simulink model "MPPT_Fuzzy"  (R2021b)
settings: Solver=ode45  StartTime=0.0  StopTime=1  FixedStep=1e-5  MaxStep=1e-4  RelTol=10e-4  EnableMultiTasking=on
libraries: spsSeriesRLCBranchLib x6, spsStairGeneratorLib x4, spsIdealSwitchLib x3, spsDiodeLib x1, fuzblock x1, powerlib_extras x1, spsGroundLib x1, spsIGBTDiodeLib x1, spsCurrentMeasurementLib x1, spsVoltageMeasurementLib x1, spsPVArrayLib x1, spsPWMGeneratorDCDCLib x1
settings Model: Creator=Administrator  LastModifiedBy=Madesh
settings SolverCC: AlgebraicLoopSolver=TrustRegion
settings DataIOCC: LimitDataPoints=on  SaveFormat=Array  SignalLoggingSaveFormat=ModelDataLogs  ReturnWorkspaceOutputs=off
settings OptimizationCC: ExpressionDepthLimit=2147483647  LifeSpan=inf
settings DebuggingCC: UnderspecifiedInitializationDetection=Classic  MergeDetectMultiDrivingBlocksExec=none  SolverPrmCheckMsg=warning  FcnCallInpInsideContextMsg=warning  StateNameClashWarn=warning  SFUnexpectedBacktrackingDiag=warning  SFNoUnconditionalDefaultTransitionDiag=warning  SFExecutionAtInitializationDiag=none  SFMachineParentedDataDiag=warning  ArithmeticOperatorsInVariantConditions=warning
settings HardwareCC: ProdBitPerPointer=32  ProdBitPerSizeT=32  ProdBitPerPtrDiffT=32  ProdLargestAtomicFloat=None  ProdIntDivRoundTo=Undefined  ProdEndianess=Unspecified  ProdWordSize=32  ProdHWDeviceType=32-bit Generic
settings ModelReferenceCC: PropagateSignalLabelsOutOfModel=off
settings SFSimCC: SimUseLocalCustomCode=off  CustomCodeUndefinedFunction=UseInterfaceOnly
settings RTWCC: RTWUseLocalCustomCode=off
settings CodeAppCC: StateflowObjectComments=on
settings GRTTargetCC: TargetLangStandard=C89/C90 (ANSI)  CombineOutputUpdateFcns=off  GRTInterface=on
settings ConfigComp: CovMetricSettings=dw  CovSaveCumulativeToWorkspaceVar=on  CovSaveSingleToWorkspaceVar=on  CovExternalEMLEnable=off
settings SimscapeCC: SimscapeNormalizeSystem=off

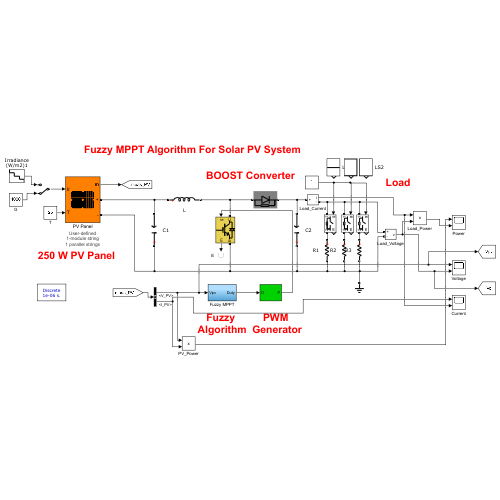
[thumbnail: Simulink's stored preview of the top-level diagram]
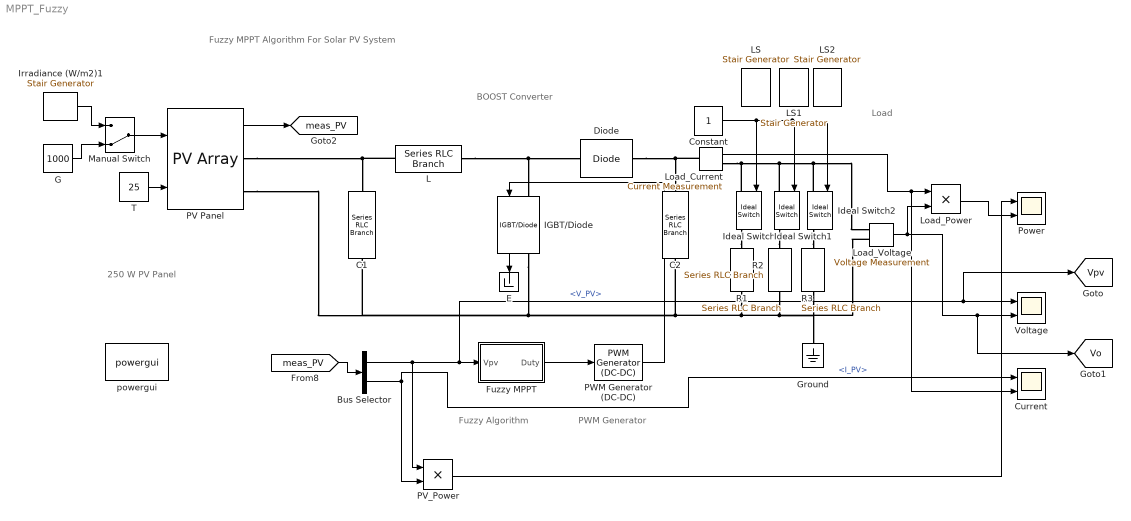
== system MPPT_Fuzzy ==
  note: Load
  note: Fuzzy MPPT Algorithm For Solar PV System
  note: BOOST Converter
  note: 250 W PV Panel
  note: Fuzzy
      | Algorithm
  note: PWM
      | Generator
  Bus Selector : BusSelector  OutputSignals=V_PV,I_PV
  C1 : spsSeriesRLCBranchLib/Series RLC Branch  LConnTagsString=__new0  RConnTagsString=__new0  BranchType=C  Resistance=1  Inductance=1e-3  SetiL0=off  InitialCurrent=0  Capacitance=100e-6  Setx0=off  InitialVoltage=0  Measurements=None
  C2 : spsSeriesRLCBranchLib/Series RLC Branch  LConnTagsString=__new0  RConnTagsString=__new0  BranchType=C  Resistance=1  Inductance=1e-3  SetiL0=off  InitialCurrent=0  Capacitance=100e-6  Setx0=off  InitialVoltage=0  Measurements=None
  Constant : Constant
  Current : Scope  NumInputPorts=2
  Diode : spsDiodeLib/Diode  Ron=0.001  Lon=0  Vf=0.8  IC=0  UseSnubber=off  Rs=500  Cs=250e-9  Measurements=off
  E : Terminator
  Fuzzy MPPT : Subsystem
  G : Constant  Value=1000
  Ground : spsGroundLib/Ground  LConnTagsString=a
  IGBT/Diode : spsIGBTDiodeLib/IGBT//Diode  Ron=1e-3  Rs=1e5  Cs=inf  Measurements=on
  Ideal Switch : spsIdealSwitchLib/Ideal Switch  Ron=0.001  Lon=0  IC=0  Rs=1e5  Cs=inf  Measurements=on
  Ideal Switch1 : spsIdealSwitchLib/Ideal Switch  Ron=0.001  Lon=0  IC=0  Rs=1e5  Cs=inf  Measurements=on
  Ideal Switch2 : spsIdealSwitchLib/Ideal Switch  Ron=0.001  Lon=0  IC=0  Rs=1e5  Cs=inf  Measurements=on
  Irradiance (W/m2)1 : spsStairGeneratorLib/Stair Generator  t=[0, 0.2 , 0.4 , 0.6, 0.8]  e=[1,0.8,0.6,0.4, 0.2]*1000  Ts=0.0001
  L : spsSeriesRLCBranchLib/Series RLC Branch  LConnTagsString=__new0  RConnTagsString=__new0  BranchType=L  Resistance=1  Inductance=3e-3  SetiL0=off  InitialCurrent=0  Capacitance=1e-6  Setx0=off  InitialVoltage=0  Measurements=None
  LS : spsStairGeneratorLib/Stair Generator  t=[0, 0.3]  e=[1, 0]  Ts=0.0001
  LS1 : spsStairGeneratorLib/Stair Generator  t=[0, 0.3, 0.6]  e=[0, 1, 0]  Ts=0.0001
  LS2 : spsStairGeneratorLib/Stair Generator  t=[0, 0.3, 0.6]  e=[0, 0, 1]  Ts=0.0001
  Load_Current : spsCurrentMeasurementLib/Current Measurement  PhasorSimulation=off  OutputType=Complex  PSBequivalent=0
  Load_Power : Product  RndMeth=Zero
  Load_Voltage : spsVoltageMeasurementLib/Voltage Measurement  PhasorSimulation=off  OutputType=Complex  PSBequivalent=0
  Manual Switch : ManualSwitch  CurrentSetting=0
  PV Panel : spsPVArrayLib/PV Array  Npar=1  Nser=1  PlotType=one module @ 25 deg.C & specified irradiances  S_vec="[ 1000 800  600  400 200 100 50]"  Temp_C_vec="[ 45 25  ]"  ModuleName=User-defined  PlotWhenSelected=off  Pm=250.205  Ncell=60  Voc=37.3  Isc=8.66  Vm=30.7  Im=8.15  beta_Voc_pc=-0.36901  alpha_Isc_pc=0.086998  beta_Voc=-0.13764  alpha_Isc=0.007534  IL=8.7062  I0=4.1579e-10  nI=1.0189  Rsh=240.6015  Rs=0.23732  RobustModel=off  RobustCellTemperature=313.3991  BAL=off  Tc=1e-6  Tfilter=1e-5
      settings: AttributesFormatString=|
      | %<ModuleName>
      | %<Nser>-module string
      | %<Npar> parallel strings
  PV_Power : Product  RndMeth=Zero
  PWM Generator (DC-DC) : spsPWMGeneratorDCDCLib/PWM Generator (DC-DC)  Fsw=10000  Ts=0
  Power : Scope  NumInputPorts=2
  R1 : spsSeriesRLCBranchLib/Series RLC Branch  LConnTagsString=__new0  RConnTagsString=__new0  BranchType=R  Resistance=20  Inductance=1e-3  SetiL0=off  InitialCurrent=0  Capacitance=1e-6  Setx0=off  InitialVoltage=0  Measurements=None
  R2 : spsSeriesRLCBranchLib/Series RLC Branch  LConnTagsString=__new0  RConnTagsString=__new0  BranchType=R  Resistance=30  Inductance=1e-3  SetiL0=off  InitialCurrent=0  Capacitance=1e-6  Setx0=off  InitialVoltage=0  Measurements=None
  R3 : spsSeriesRLCBranchLib/Series RLC Branch  LConnTagsString=__new0  RConnTagsString=__new0  BranchType=R  Resistance=60  Inductance=1e-3  SetiL0=off  InitialCurrent=0  Capacitance=1e-6  Setx0=off  InitialVoltage=0  Measurements=None
  T : Constant  Value=25
  Voltage : Scope  NumInputPorts=2
  powergui : spspowerguiLib/powergui  Priority=1  SimulationMode=Discrete  SampleTime=1e-6  frequency=60  Iterations=50  frequencyindice=0  Pbase=100e6  ErrMax=1e-4  UnitsV=kV  UnitsW=MW  buscounter=0  FunctionMessages=off  echomessages=off  EnableUseOfTLC=off  CurrentSourceSwitches=off  DisableSnubberDevices=off  DisableRonSwitches=off  DisableVfSwitches=off  DisplayEquations=off  AutomaticDiscreteSolvers=off  SolverType=Tustin/Backward Euler (TBE)  Interpol=off  ExternalGateDelay=off  methode=off  Ts=100  x0status=blocks  SPID=on  SwTol=0  HookPort=off  NonlinearTolerance=1e-4  nMaxIteration=100  ContinueOnMaxIteration=off  RestoreLinks=warning  ResistiveCurrentMeasurement=off  Frange=[0:2:500]  Ylog=off  Xlog=on  ShowGrid=off  save=off  variable=ZData  structure=0  ZoomFFT=off  StartTime=0.0  cycles=1  DisplayStyle=1  fundamental=60  FreqAxis=off  MaxFrequency=1000  frequencyindicesteady=1  RmsSteady=1  display=off
  tag scope: Vo=global, Vpv=global, meas_PV=global
  wires:
  T/1 -> PV Panel/2
  IGBT/Diode/1 -> E/1
  PV Panel/1 -> [meas_PV]
  [meas_PV] -> Bus Selector/1
  Bus Selector/2 -> Current/1, PV_Power/2  "<I_PV>"
  Bus Selector/1 -> [Vpv], Voltage/1, Fuzzy MPPT/1(Vpv), PV_Power/1  "<V_PV>"
  Load_Voltage/1 -> [Vo], Voltage/2, Load_Power/2
  Load_Current/1 -> Current/2, Load_Power/1
  Load_Power/1 -> Power/2
  PV_Power/1 -> Power/1
  Manual Switch/1 -> PV Panel/1
  Irradiance (W/m2)1/1 -> Manual Switch/1
  G/1 -> Manual Switch/2
  PWM Generator (DC-DC)/1 -> IGBT/Diode/1
  Fuzzy MPPT/1(Duty) -> PWM Generator (DC-DC)/1
  Constant/1 -> Ideal Switch1/1, Ideal Switch2/1, Ideal Switch/1
  connections:
  L/LConn1 -- PV Panel/RConn1 -- C1/RConn1
  L/RConn1 -- Diode/LConn1 -- IGBT/Diode/LConn1
  R2/RConn1 -- Ground/LConn1 -- Load_Voltage/LConn2 -- R3/RConn1 -- R1/RConn1 -- C2/LConn1 -- PV Panel/RConn2 -- C1/LConn1 -- IGBT/Diode/RConn1
  Diode/RConn1 -- Load_Current/LConn1 -- C2/RConn1
  Load_Current/RConn1 -- Ideal Switch2/LConn1 -- Load_Voltage/LConn1 -- Ideal Switch1/LConn1 -- Ideal Switch/LConn1
  Ideal Switch/RConn1 -- R1/LConn1
  Ideal Switch1/RConn1 -- R2/LConn1
  Ideal Switch2/RConn1 -- R3/LConn1

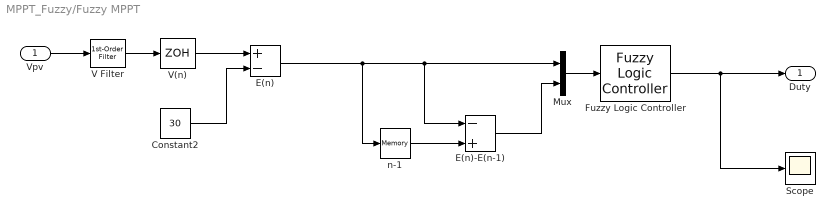
== system MPPT_Fuzzy/Fuzzy MPPT ==
  Vpv : Inport
  Constant2 : Constant  Value=30
  E(n) : Sum  Inputs=+-
  E(n)-E(n-1) : Sum  Inputs=-+
  Fuzzy Logic Controller : fuzblock/Fuzzy Logic  Controller  FIS='flc.fis'  OutputSampleNumber=101  DataType=double  FuzzifiedInputs=off  RuleFiringStrengths=off  RuleOutputs=off  AggregatedOutputs=off  SimulateUsing=Interpreted execution  OutOfRangeInputValueMessage=warning  NoRuleFiredMessage=warning  EmptyOutputFuzzySetMessage=warning
  Mux : Mux  Inputs=2
  Scope : Scope
  V Filter : powerlib_extras/Control  Blocks/1st-Order  Filter  FilterType=Lowpass  Tc=30e-3  Initialize=off  Vac_Init=[0.8 -25 60]  Vdc_Init=-0.4  PlotResponse=off  param1=[1 500 1]
      settings: SourceProductBaseCode=PS
  V(n) : ZeroOrderHold  SampleTime=1e-4
  n-1 : Memory  InheritSampleTime=on  LinearizeAsDelay=on
  Duty : Outport  VectorParamsAs1DForOutWhenUnconnected=off
  wires:
  Vpv/1 -> V Filter/1
  V Filter/1 -> V(n)/1
  Mux/1 -> Fuzzy Logic Controller/1
  V(n)/1 -> E(n)/1
  Constant2/1 -> E(n)/2
  E(n)-E(n-1)/1 -> Mux/2
  n-1/1 -> E(n)-E(n-1)/2
  Fuzzy Logic Controller/1 -> Scope/1, Duty/1
  E(n)/1 -> Mux/1, E(n)-E(n-1)/1, n-1/1
